simulink model "Linear_model_Kalman_Bucy"  (R2025b)
settings: Solver=VariableStepAuto  StartTime=0.0  StopTime=10.0  RelTol=1e-3
values from neighbouring files (symbols this model uses):
  A1 = [0, 1; 0, 0]    [ABCDmatrixes_for_linear.m]    (also in drone_model_parameters.mat = [0  1; 0  0]; kalman_observer_linear_Q9_RUN_THIS.m)
  A2 = [0, 0, 1, 0; 0, 0, 0, 1; 0, g, 0, 0; 0, 0, 0, 0]    [ABCDmatrixes_for_linear.m]    (also in drone_model_parameters.mat = [0 0 0 0 0 0 9.81 0 1 0 0 0 ... (16 elements, 4x4)]; kalman_observer_linear_Q9_RUN_THIS.m)
  A3 = [0, 0, 1, 0; 0, 0, 0, 1; 0, -g, 0, 0; 0, 0, 0, 0]    [ABCDmatrixes_for_linear.m]    (also in drone_model_parameters.mat = [0 0 0 0 0 0 -9.81 0 1 0 0 0 ... (16 elements, 4x4)]; kalman_observer_linear_Q9_RUN_THIS.m)
  A4 = [0, 1; 0, 0]    [ABCDmatrixes_for_linear.m]    (also in drone_model_parameters.mat = [0  1; 0  0]; kalman_observer_linear_Q9_RUN_THIS.m)
  B1 = [0; 1/m]    [ABCDmatrixes_for_linear.m]    (also in drone_model_parameters.mat = [0 15.873015873]; kalman_observer_linear_Q9_RUN_THIS.m)
  B2 = [0; 0; 0; 1/J11]    [ABCDmatrixes_for_linear.m]    (also in drone_model_parameters.mat = [0 0 0 17156.7786432]; kalman_observer_linear_Q9_RUN_THIS.m)
  B3 = [0; 0; 0; 1/J22]    [ABCDmatrixes_for_linear.m]    (also in drone_model_parameters.mat = [0 0 0 13948.7522841]; kalman_observer_linear_Q9_RUN_THIS.m)
  B4 = [0; 1/J33]    [ABCDmatrixes_for_linear.m]    (also in drone_model_parameters.mat = [0 33333.3333333]; kalman_observer_linear_Q9_RUN_THIS.m)
  C1 = eye(2)    [ABCDmatrixes_for_linear.m]    (also in drone_model_parameters.mat = [1  0; 0  1]; kalman_observer_linear_Q9_RUN_THIS.m)
  C2 = eye(4)    [ABCDmatrixes_for_linear.m]    (also in drone_model_parameters.mat = [1 0 0 0 0 1 0 0 0 0 1 0 ... (16 elements, 4x4)]; kalman_observer_linear_Q9_RUN_THIS.m)
  C3 = eye(4)    [ABCDmatrixes_for_linear.m]    (also in drone_model_parameters.mat = [1 0 0 0 0 1 0 0 0 0 1 0 ... (16 elements, 4x4)]; kalman_observer_linear_Q9_RUN_THIS.m)
  C4 = eye(2)    [ABCDmatrixes_for_linear.m]    (also in drone_model_parameters.mat = [1  0; 0  1]; kalman_observer_linear_Q9_RUN_THIS.m)
  K1 = [0.567 0.2646]    [drone_model_parameters.mat]    (also in kalman_observer_linear_Q9_RUN_THIS.m = place(A1, B1, poles1); lqr_servo_controller.m = K1_lqr(1:2))
  K2 = [0.00422225922936 0.00948429792 0.00292221406239 0.001282292]    [drone_model_parameters.mat]    (also in kalman_observer_linear_Q9_RUN_THIS.m = place(A2, B2, poles2); lqr_servo_controller.m = K2_lqr(1:4))
  K3 = [-0.00519332234862 0.01166555952 -0.00359428419083 0.001577202]    [drone_model_parameters.mat]    (also in kalman_observer_linear_Q9_RUN_THIS.m = place(A3, B3, poles3); lqr_servo_controller.m = K3_lqr(1:4))
  K4 = [0.00015 0.000135]    [drone_model_parameters.mat]    (also in kalman_observer_linear_Q9_RUN_THIS.m = place(A4, B4, poles4); lqr_servo_controller.m = K4_lqr(1:2))
  ki1 = 0.567    [drone_model_parameters.mat]    (also in kalman_observer_linear_Q9_RUN_THIS.m = prefilter(A1, B1, C1(1,:), K1); lqr_servo_controller.m = -K1_lqr(3))
  ki2 = 0.00422225922936    [drone_model_parameters.mat]    (also in kalman_observer_linear_Q9_RUN_THIS.m = prefilter(A2, B2, C2(1,:), K2); lqr_servo_controller.m = -K2_lqr(5))
  ki3 = -0.00519332234862    [drone_model_parameters.mat]    (also in kalman_observer_linear_Q9_RUN_THIS.m = prefilter(A3, B3, C3(1,:), K3); lqr_servo_controller.m = -K3_lqr(5))
  ki4 = 0.00015    [drone_model_parameters.mat]    (also in kalman_observer_linear_Q9_RUN_THIS.m = prefilter(A4, B4, C4(1,:), K4); lqr_servo_controller.m = -K4_lqr(3))
  L1 = [7.45658027326  0.497973338958; 0.0505189943149  7.39637645576]    [drone_model_parameters.mat]
  L2 = [1.45150777342 2.3802958397e-05 0.00454213306172 -1.52026813527e-09 0.0292749657214 29.2123228098 7.26957664981 0.00232988214846 0.87651500602 1.14062573329 10.208521833 2.76371424964e-05 ... (16 elements, 4x4)]    [drone_model_parameters.mat]
  L3 = [1.11002532922 -8.8269645689e-06 0.00273068540644 1.79452583191e-09 -0.0248011961907 27.5933010049 -7.19451191698 0.00571707644971 0.901052348557 -0.844925554559 10.0312929821 -6.86940481085e-05 ... (16 elements, 4x4)]    [drone_model_parameters.mat]
  L4 = [1.61563059299  0.880343962343; 0.000162624550244  11.8866600113]    [drone_model_parameters.mat]
  noise_P_lat = [0.009 0.003 0.002 1e-05]    [drone_model_parameters.mat]    (also in kalman_observer_linear_Q9_RUN_THIS.m = [var_P_r2,  var_P_th1, var_P_v2,  var_P_om1] * Ts)
  noise_P_lon = [0.009 0.002 0.002 1e-05]    [drone_model_parameters.mat]    (also in kalman_observer_linear_Q9_RUN_THIS.m = [var_P_r1,  var_P_th2, var_P_v1,  var_P_om2] * Ts)
  noise_P_vert = [0.001 0.0001]    [drone_model_parameters.mat]    (also in kalman_observer_linear_Q9_RUN_THIS.m = [var_P_r3,  var_P_v3]  * Ts)
  noise_P_yaw = [0.001 1e-05]    [drone_model_parameters.mat]    (also in kalman_observer_linear_Q9_RUN_THIS.m = [var_P_th3, var_P_om3] * Ts)
  phi_ref = 1    [drone_model_parameters.mat]    (also in kalman_observer_linear_Q9_RUN_THIS.m)
  Ts = 0.01    [drone_model_parameters.mat]    (also in kalman_observer_linear_Q9_RUN_THIS.m)
  x0_1 = [0 0]    [drone_model_parameters.mat]    (also in kalman_observer_linear_Q9_RUN_THIS.m = [0; 0])
  x0_2 = [0 0 0 0]    [drone_model_parameters.mat]    (also in kalman_observer_linear_Q9_RUN_THIS.m = [0; 0; 0; 0])
  x0_3 = [0 0 0 0]    [drone_model_parameters.mat]    (also in kalman_observer_linear_Q9_RUN_THIS.m = [0; 0; 0; 0])
  x0_4 = [0 0]    [drone_model_parameters.mat]    (also in kalman_observer_linear_Q9_RUN_THIS.m = [0; 0])
  x0_obs1 = [0 0]    [drone_model_parameters.mat]    (also in kalman_observer_linear_Q9_RUN_THIS.m = [0; 0])
  x0_obs2 = [0 0 0 0]    [drone_model_parameters.mat]    (also in kalman_observer_linear_Q9_RUN_THIS.m = [0; 0; 0; 0])
  x0_obs3 = [0 0 0 0]    [drone_model_parameters.mat]    (also in kalman_observer_linear_Q9_RUN_THIS.m = [0; 0; 0; 0])
  x0_obs4 = [0 0]    [drone_model_parameters.mat]    (also in kalman_observer_linear_Q9_RUN_THIS.m = [0; 0])
  x_ref = 4    [drone_model_parameters.mat]    (also in kalman_observer_linear_Q9_RUN_THIS.m)
  y_ref = 4    [drone_model_parameters.mat]    (also in kalman_observer_linear_Q9_RUN_THIS.m)
  z_ref = 4    [drone_model_parameters.mat]    (also in kalman_observer_linear_Q9_RUN_THIS.m)
libraries: simulink x8
settings Model: Creator=joaom  LastModifiedBy=pepev
settings DataIOCC: SaveFormat=Array

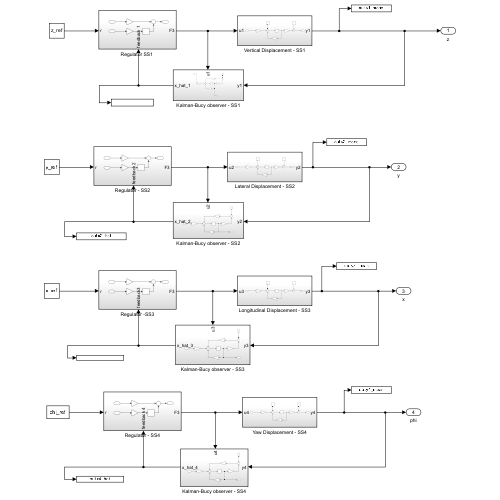
[thumbnail: Simulink's stored preview of the top-level diagram]
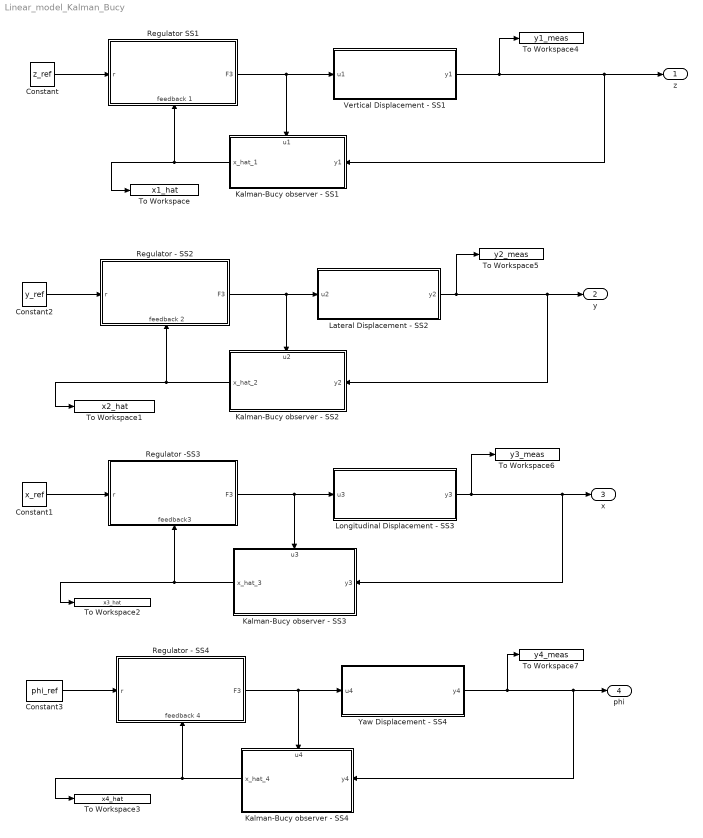
== system Linear_model_Kalman_Bucy ==
  Constant : Constant  Value=z_ref
  Constant1 : Constant  Value=x_ref
  Constant2 : Constant  Value=y_ref
  Constant3 : Constant  Value=phi_ref
  Kalman-Bucy observer - SS1 : Subsystem
      settings: PortSchema="{\"entries\":[{\"content\":{\"sides\":[{\"content\":{\"connectorIds\":[\"Out1\"]},\"type\":\"ConnectorPlacement.EquallySpacedRectSide\",\"uuid\":\"3a34d9e3-ef6b-4e0e-ad1c-a8e9abb9cb50\"},{\"content\":{\"connectorIds\":[\"In2\"],\"side\":\"RIGHT\"},\"type\":\"ConnectorPlacement.EquallySpacedRectSide\",\"uuid\":\"1b685036-9c62-4d8c-a792-6e44f47fda20\"},{\"content\":{\"connectorIds\":[\"In1\"],\"side\":\"TOP\"},\"type\":\"ConnectorPlacement.EquallySpacedRectSide\",\"uuid\":\"5c00f917-5739-44a5-95b0-e7bd6f61a97f\"}]},\"type\":\"ConnectorPlacement.EquallySpacedConnector\",\"uuid\":\"e365f2b2-c96f-4048-9751-de98e4d7538e\"}],\"packageUris\":[\"http://schema.mathworks.com/mf0/Connector/R2020b\"],\"version\":\"1.0\"}"
  Kalman-Bucy observer - SS2 : Subsystem
      settings: PortSchema="{\"entries\":[{\"content\":{\"sides\":[{\"content\":{\"connectorIds\":[\"Out1\"]},\"type\":\"ConnectorPlacement.EquallySpacedRectSide\",\"uuid\":\"3a34d9e3-ef6b-4e0e-ad1c-a8e9abb9cb50\"},{\"content\":{\"connectorIds\":[\"In2\"],\"side\":\"RIGHT\"},\"type\":\"ConnectorPlacement.EquallySpacedRectSide\",\"uuid\":\"1b685036-9c62-4d8c-a792-6e44f47fda20\"},{\"content\":{\"connectorIds\":[\"In1\"],\"side\":\"TOP\"},\"type\":\"ConnectorPlacement.EquallySpacedRectSide\",\"uuid\":\"5c00f917-5739-44a5-95b0-e7bd6f61a97f\"}]},\"type\":\"ConnectorPlacement.EquallySpacedConnector\",\"uuid\":\"e365f2b2-c96f-4048-9751-de98e4d7538e\"}],\"packageUris\":[\"http://schema.mathworks.com/mf0/Connector/R2020b\"],\"version\":\"1.0\"}"
  Kalman-Bucy observer - SS3 : Subsystem
      settings: PortSchema="{\"entries\":[{\"content\":{\"sides\":[{\"content\":{\"connectorIds\":[\"Out1\"]},\"type\":\"ConnectorPlacement.EquallySpacedRectSide\",\"uuid\":\"3a34d9e3-ef6b-4e0e-ad1c-a8e9abb9cb50\"},{\"content\":{\"connectorIds\":[\"In2\"],\"side\":\"RIGHT\"},\"type\":\"ConnectorPlacement.EquallySpacedRectSide\",\"uuid\":\"1b685036-9c62-4d8c-a792-6e44f47fda20\"},{\"content\":{\"connectorIds\":[\"In1\"],\"side\":\"TOP\"},\"type\":\"ConnectorPlacement.EquallySpacedRectSide\",\"uuid\":\"5c00f917-5739-44a5-95b0-e7bd6f61a97f\"}]},\"type\":\"ConnectorPlacement.EquallySpacedConnector\",\"uuid\":\"e365f2b2-c96f-4048-9751-de98e4d7538e\"}],\"packageUris\":[\"http://schema.mathworks.com/mf0/Connector/R2020b\"],\"version\":\"1.0\"}"
  Kalman-Bucy observer - SS4 : Subsystem
      settings: PortSchema="{\"entries\":[{\"content\":{\"sides\":[{\"content\":{\"connectorIds\":[\"Out1\"]},\"type\":\"ConnectorPlacement.EquallySpacedRectSide\",\"uuid\":\"3a34d9e3-ef6b-4e0e-ad1c-a8e9abb9cb50\"},{\"content\":{\"connectorIds\":[\"In2\"],\"side\":\"RIGHT\"},\"type\":\"ConnectorPlacement.EquallySpacedRectSide\",\"uuid\":\"1b685036-9c62-4d8c-a792-6e44f47fda20\"},{\"content\":{\"connectorIds\":[\"In1\"],\"side\":\"TOP\"},\"type\":\"ConnectorPlacement.EquallySpacedRectSide\",\"uuid\":\"5c00f917-5739-44a5-95b0-e7bd6f61a97f\"}]},\"type\":\"ConnectorPlacement.EquallySpacedConnector\",\"uuid\":\"e365f2b2-c96f-4048-9751-de98e4d7538e\"}],\"packageUris\":[\"http://schema.mathworks.com/mf0/Connector/R2020b\"],\"version\":\"1.0\"}"
  Lateral Displacement - SS2 : Subsystem
  Longitudinal Displacement - SS3 : Subsystem
  Regulator - SS2 : Subsystem
      settings: PortSchema="{\"entries\":[{\"content\":{\"sides\":[{\"content\":{\"connectorIds\":[\"In1\"]},\"type\":\"ConnectorPlacement.EquallySpacedRectSide\",\"uuid\":\"b3654a7f-5063-48c0-9b36-91e0db63b0ba\"},{\"content\":{\"connectorIds\":[\"Out1\"],\"side\":\"RIGHT\"},\"type\":\"ConnectorPlacement.EquallySpacedRectSide\",\"uuid\":\"218488d6-68f2-41aa-8299-f3fb09ba40d8\"},{\"content\":{\"side\":\"TOP\"},\"type\":\"ConnectorPlacement.EquallySpacedRectSide\",\"uuid\":\"ffca8f5f-99ce-4cfe-b848-505d5918397a\"},{\"content\":{\"connectorIds\":[\"In2\"],\"side\":\"BOTTOM\"},\"type\":\"ConnectorPlacement.EquallySpacedRectSide\",\"uuid\":\"0ee1b0b7-fa1d-4d2f-b721-1db90edeb8b7\"}]},\"type\":\"ConnectorPlacement.EquallySpacedConnector\",\"uuid\":\"97e1b17e-acc2-4e54-bcf8-8316abbe6834\"}],\"packageUris\":[\"http://schema.mathworks.com/mf0/Connector/R2020b\"],\"version\":\"1.0\"}"
  Regulator - SS4 : Subsystem
      settings: PortSchema="{\"entries\":[{\"content\":{\"sides\":[{\"content\":{\"connectorIds\":[\"In1\"]},\"type\":\"ConnectorPlacement.EquallySpacedRectSide\",\"uuid\":\"b3654a7f-5063-48c0-9b36-91e0db63b0ba\"},{\"content\":{\"connectorIds\":[\"Out1\"],\"side\":\"RIGHT\"},\"type\":\"ConnectorPlacement.EquallySpacedRectSide\",\"uuid\":\"218488d6-68f2-41aa-8299-f3fb09ba40d8\"},{\"content\":{\"side\":\"TOP\"},\"type\":\"ConnectorPlacement.EquallySpacedRectSide\",\"uuid\":\"ffca8f5f-99ce-4cfe-b848-505d5918397a\"},{\"content\":{\"connectorIds\":[\"In2\"],\"side\":\"BOTTOM\"},\"type\":\"ConnectorPlacement.EquallySpacedRectSide\",\"uuid\":\"0ee1b0b7-fa1d-4d2f-b721-1db90edeb8b7\"}]},\"type\":\"ConnectorPlacement.EquallySpacedConnector\",\"uuid\":\"97e1b17e-acc2-4e54-bcf8-8316abbe6834\"}],\"packageUris\":[\"http://schema.mathworks.com/mf0/Connector/R2020b\"],\"version\":\"1.0\"}"
  Regulator -SS3 : Subsystem
      settings: PortSchema="{\"entries\":[{\"content\":{\"sides\":[{\"content\":{\"connectorIds\":[\"In1\"]},\"type\":\"ConnectorPlacement.EquallySpacedRectSide\",\"uuid\":\"b3654a7f-5063-48c0-9b36-91e0db63b0ba\"},{\"content\":{\"connectorIds\":[\"Out1\"],\"side\":\"RIGHT\"},\"type\":\"ConnectorPlacement.EquallySpacedRectSide\",\"uuid\":\"218488d6-68f2-41aa-8299-f3fb09ba40d8\"},{\"content\":{\"side\":\"TOP\"},\"type\":\"ConnectorPlacement.EquallySpacedRectSide\",\"uuid\":\"ffca8f5f-99ce-4cfe-b848-505d5918397a\"},{\"content\":{\"connectorIds\":[\"In2\"],\"side\":\"BOTTOM\"},\"type\":\"ConnectorPlacement.EquallySpacedRectSide\",\"uuid\":\"0ee1b0b7-fa1d-4d2f-b721-1db90edeb8b7\"}]},\"type\":\"ConnectorPlacement.EquallySpacedConnector\",\"uuid\":\"97e1b17e-acc2-4e54-bcf8-8316abbe6834\"}],\"packageUris\":[\"http://schema.mathworks.com/mf0/Connector/R2020b\"],\"version\":\"1.0\"}"
  "Regulator SS1 " : Subsystem
      settings: PortSchema="{\"entries\":[{\"content\":{\"sides\":[{\"content\":{\"connectorIds\":[\"In1\"]},\"type\":\"ConnectorPlacement.EquallySpacedRectSide\",\"uuid\":\"b3654a7f-5063-48c0-9b36-91e0db63b0ba\"},{\"content\":{\"connectorIds\":[\"Out1\"],\"side\":\"RIGHT\"},\"type\":\"ConnectorPlacement.EquallySpacedRectSide\",\"uuid\":\"218488d6-68f2-41aa-8299-f3fb09ba40d8\"},{\"content\":{\"side\":\"TOP\"},\"type\":\"ConnectorPlacement.EquallySpacedRectSide\",\"uuid\":\"ffca8f5f-99ce-4cfe-b848-505d5918397a\"},{\"content\":{\"connectorIds\":[\"In2\"],\"side\":\"BOTTOM\"},\"type\":\"ConnectorPlacement.EquallySpacedRectSide\",\"uuid\":\"0ee1b0b7-fa1d-4d2f-b721-1db90edeb8b7\"}]},\"type\":\"ConnectorPlacement.EquallySpacedConnector\",\"uuid\":\"97e1b17e-acc2-4e54-bcf8-8316abbe6834\"}],\"packageUris\":[\"http://schema.mathworks.com/mf0/Connector/R2020b\"],\"version\":\"1.0\"}"
  To Workspace : ToWorkspace  VariableName=x1_hat  SampleTime=-1
  To Workspace1 : ToWorkspace  VariableName=x2_hat  SampleTime=-1
  To Workspace2 : ToWorkspace  VariableName=x3_hat  SampleTime=-1
  To Workspace3 : ToWorkspace  VariableName=x4_hat  SampleTime=-1
  To Workspace4 : ToWorkspace  VariableName=y1_meas  SampleTime=-1
  To Workspace5 : ToWorkspace  VariableName=y2_meas  SampleTime=-1
  To Workspace6 : ToWorkspace  VariableName=y3_meas  SampleTime=-1
  To Workspace7 : ToWorkspace  VariableName=y4_meas  SampleTime=-1
  Vertical Displacement - SS1 : Subsystem
  Yaw Displacement - SS4 : Subsystem
  z : Outport
  y : Outport  Port=2
  x : Outport  Port=3
  phi : Outport  Port=4
  wires:
  Constant/1 -> "Regulator SS1 "/1(r)
  "Regulator SS1 "/1(F3) -> Kalman-Bucy observer - SS1/1(u1), Vertical Displacement - SS1/1(u1)
  Constant2/1 -> Regulator - SS2/1(r)
  Regulator - SS2/1(F3) -> Kalman-Bucy observer - SS2/1(u2), Lateral Displacement - SS2/1(u2)
  Constant1/1 -> Regulator -SS3/1(r)
  Regulator -SS3/1(F3) -> Longitudinal Displacement - SS3/1(u3), Kalman-Bucy observer - SS3/1(u3)
  Yaw Displacement - SS4/1(y4) -> To Workspace7/1, Kalman-Bucy observer - SS4/2(y4), phi/1
  Constant3/1 -> Regulator - SS4/1(r)
  Regulator - SS4/1(F3) -> Kalman-Bucy observer - SS4/1(u4), Yaw Displacement - SS4/1(u4)
  Kalman-Bucy observer - SS1/1(x_hat_1) -> To Workspace/1, "Regulator SS1 "/2(feedback 1)
  Kalman-Bucy observer - SS3/1(x_hat_3) -> To Workspace2/1, Regulator -SS3/2(feedback3)
  Kalman-Bucy observer - SS4/1(x_hat_4) -> To Workspace3/1, Regulator - SS4/2(feedback 4)
  Kalman-Bucy observer - SS2/1(x_hat_2) -> Regulator - SS2/2(feedback 2), To Workspace1/1
  Vertical Displacement - SS1/1(y1) -> Kalman-Bucy observer - SS1/2(y1), z/1, To Workspace4/1
  Lateral Displacement - SS2/1(y2) -> To Workspace5/1, Kalman-Bucy observer - SS2/2(y2), y/1
  Longitudinal Displacement - SS3/1(y3) -> To Workspace6/1, Kalman-Bucy observer - SS3/2(y3), x/1

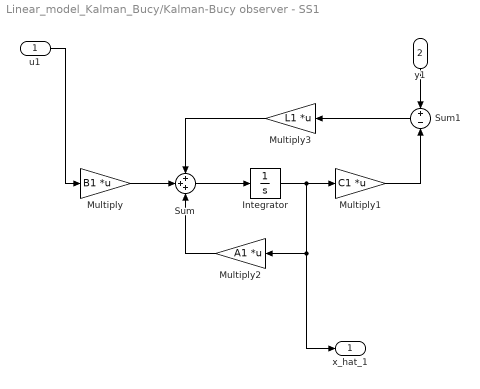
== system Linear_model_Kalman_Bucy/Kalman-Bucy observer - SS1 ==
  u1 : Inport
  y1 : Inport  Port=2
  Integrator : Integrator  InitialCondition=x0_obs1
  Multiply : Gain  Gain=B1  Multiplication=Matrix(K*u)
  Multiply1 : Gain  Gain=C1  Multiplication=Matrix(K*u)
  Multiply2 : Gain  Gain=A1  Multiplication=Matrix(K*u)
  Multiply3 : Gain  Gain=L1  Multiplication=Matrix(K*u)
  Sum : Sum  Inputs=+++
  Sum1 : Sum  Inputs=+|-
  x_hat_1 : Outport
  wires:
  Multiply2/1 -> Sum/3
  Sum/1 -> Integrator/1
  Integrator/1 -> x_hat_1/1, Multiply2/1, Multiply1/1
  u1/1 -> Multiply/1
  Multiply3/1 -> Sum/1
  Multiply/1 -> Sum/2
  Multiply1/1 -> Sum1/2
  y1/1 -> Sum1/1
  Sum1/1 -> Multiply3/1

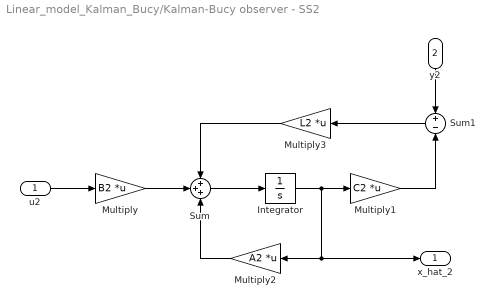
== system Linear_model_Kalman_Bucy/Kalman-Bucy observer - SS2 ==
  u2 : Inport
  y2 : Inport  Port=2
  Integrator : Integrator  InitialCondition=x0_obs2
  Multiply : Gain  Gain=B2  Multiplication=Matrix(K*u)
  Multiply1 : Gain  Gain=C2  Multiplication=Matrix(K*u)
  Multiply2 : Gain  Gain=A2  Multiplication=Matrix(K*u)
  Multiply3 : Gain  Gain=L2  Multiplication=Matrix(K*u)
  Sum : Sum  Inputs=+++
  Sum1 : Sum  Inputs=+|-
  x_hat_2 : Outport
  wires:
  Multiply2/1 -> Sum/3
  Sum/1 -> Integrator/1
  Integrator/1 -> x_hat_2/1, Multiply2/1, Multiply1/1
  u2/1 -> Multiply/1
  Multiply3/1 -> Sum/1
  Multiply/1 -> Sum/2
  Multiply1/1 -> Sum1/2
  y2/1 -> Sum1/1
  Sum1/1 -> Multiply3/1

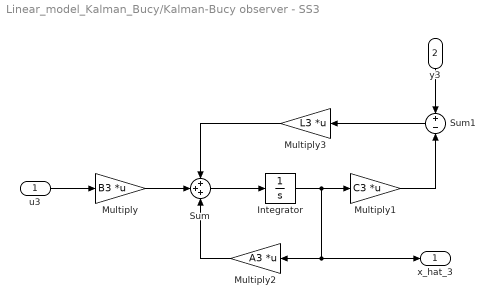
== system Linear_model_Kalman_Bucy/Kalman-Bucy observer - SS3 ==
  u3 : Inport
  y3 : Inport  Port=2
  Integrator : Integrator  InitialCondition=x0_obs3
  Multiply : Gain  Gain=B3  Multiplication=Matrix(K*u)
  Multiply1 : Gain  Gain=C3  Multiplication=Matrix(K*u)
  Multiply2 : Gain  Gain=A3  Multiplication=Matrix(K*u)
  Multiply3 : Gain  Gain=L3  Multiplication=Matrix(K*u)
  Sum : Sum  Inputs=+++
  Sum1 : Sum  Inputs=+|-
  x_hat_3 : Outport
  wires:
  Multiply2/1 -> Sum/3
  Sum/1 -> Integrator/1
  Integrator/1 -> x_hat_3/1, Multiply2/1, Multiply1/1
  u3/1 -> Multiply/1
  Multiply3/1 -> Sum/1
  Multiply/1 -> Sum/2
  Multiply1/1 -> Sum1/2
  y3/1 -> Sum1/1
  Sum1/1 -> Multiply3/1

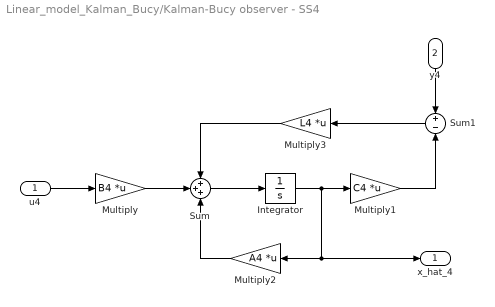
== system Linear_model_Kalman_Bucy/Kalman-Bucy observer - SS4 ==
  u4 : Inport
  y4 : Inport  Port=2
  Integrator : Integrator  InitialCondition=x0_obs4
  Multiply : Gain  Gain=B4  Multiplication=Matrix(K*u)
  Multiply1 : Gain  Gain=C4  Multiplication=Matrix(K*u)
  Multiply2 : Gain  Gain=A4  Multiplication=Matrix(K*u)
  Multiply3 : Gain  Gain=L4  Multiplication=Matrix(K*u)
  Sum : Sum  Inputs=+++
  Sum1 : Sum  Inputs=+|-
  x_hat_4 : Outport
  wires:
  Multiply2/1 -> Sum/3
  Sum/1 -> Integrator/1
  Integrator/1 -> x_hat_4/1, Multiply2/1, Multiply1/1
  u4/1 -> Multiply/1
  Multiply3/1 -> Sum/1
  Multiply/1 -> Sum/2
  Multiply1/1 -> Sum1/2
  y4/1 -> Sum1/1
  Sum1/1 -> Multiply3/1

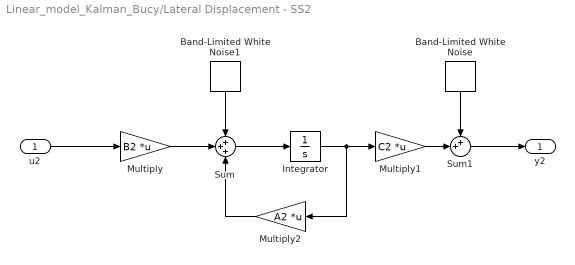
== system Linear_model_Kalman_Bucy/Lateral Displacement - SS2 ==
  u2 : Inport
  Band-Limited White Noise : simulink/Sources/Band-Limited White Noise  Cov=noise_M_lat  Ts=0.01  seed=[50 51 52 53]
  Band-Limited White Noise1 : simulink/Sources/Band-Limited White Noise  Cov=[noise_P_lat]  Ts=0.01  seed=[46 47 48 49]
  Integrator : Integrator  InitialCondition=x0_2
  Multiply : Gain  Gain=B2  Multiplication=Matrix(K*u)
  Multiply1 : Gain  Gain=C2  Multiplication=Matrix(K*u)
  Multiply2 : Gain  Gain=A2  Multiplication=Matrix(K*u)
  Sum : Sum  Inputs=+++
  Sum1 : Sum  Inputs=++|
  y2 : Outport
  wires:
  u2/1 -> Multiply/1
  Multiply/1 -> Sum/2
  Sum/1 -> Integrator/1
  Integrator/1 -> Multiply2/1, Multiply1/1
  Multiply1/1 -> Sum1/2
  Sum1/1 -> y2/1
  Multiply2/1 -> Sum/3
  Band-Limited White Noise/1 -> Sum1/1
  Band-Limited White Noise1/1 -> Sum/1

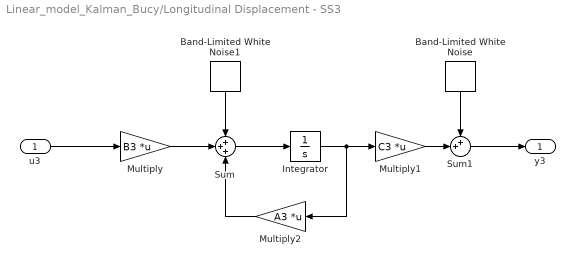
== system Linear_model_Kalman_Bucy/Longitudinal Displacement - SS3 ==
  u3 : Inport
  Band-Limited White Noise : simulink/Sources/Band-Limited White Noise  Cov=noise_M_lon  Ts=0.01  seed=[58 59 60 61]
  Band-Limited White Noise1 : simulink/Sources/Band-Limited White Noise  Cov=[noise_P_lon]  Ts=0.01  seed=[54 55 56 57]
  Integrator : Integrator  InitialCondition=x0_3
  Multiply : Gain  Gain=B3  Multiplication=Matrix(K*u)
  Multiply1 : Gain  Gain=C3  Multiplication=Matrix(K*u)
  Multiply2 : Gain  Gain=A3  Multiplication=Matrix(K*u)
  Sum : Sum  Inputs=+++
  Sum1 : Sum  Inputs=++|
  y3 : Outport
  wires:
  u3/1 -> Multiply/1
  Multiply/1 -> Sum/2
  Sum/1 -> Integrator/1
  Integrator/1 -> Multiply2/1, Multiply1/1
  Multiply1/1 -> Sum1/2
  Sum1/1 -> y3/1
  Multiply2/1 -> Sum/3
  Band-Limited White Noise/1 -> Sum1/1
  Band-Limited White Noise1/1 -> Sum/1

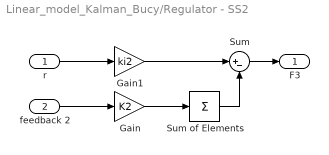
== system Linear_model_Kalman_Bucy/Regulator - SS2 ==
  r : Inport
  feedback 2 : Inport  Port=2
  Gain : Gain  Gain=K2
  Gain1 : Gain  Gain=ki2
  Sum : Sum  Inputs=|+-
  Sum of Elements : Sum  Inputs=+
  F3 : Outport
  wires:
  r/1 -> Gain1/1
  Gain1/1 -> Sum/1
  Sum/1 -> F3/1
  feedback 2/1 -> Gain/1
  Gain/1 -> Sum of Elements/1
  Sum of Elements/1 -> Sum/2

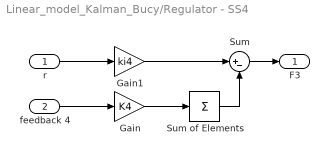
== system Linear_model_Kalman_Bucy/Regulator - SS4 ==
  r : Inport
  feedback 4 : Inport  Port=2
  Gain : Gain  Gain=K4
  Gain1 : Gain  Gain=ki4
  Sum : Sum  Inputs=|+-
  Sum of Elements : Sum  Inputs=+
  F3 : Outport
  wires:
  r/1 -> Gain1/1
  Gain1/1 -> Sum/1
  Sum/1 -> F3/1
  feedback 4/1 -> Gain/1
  Gain/1 -> Sum of Elements/1
  Sum of Elements/1 -> Sum/2

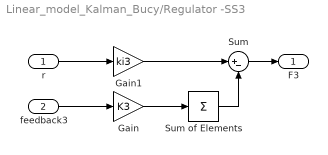
== system Linear_model_Kalman_Bucy/Regulator -SS3 ==
  r : Inport
  feedback3 : Inport  Port=2
  Gain : Gain  Gain=K3
  Gain1 : Gain  Gain=ki3
  Sum : Sum  Inputs=|+-
  Sum of Elements : Sum  Inputs=+
  F3 : Outport
  wires:
  r/1 -> Gain1/1
  Gain1/1 -> Sum/1
  Sum/1 -> F3/1
  feedback3/1 -> Gain/1
  Gain/1 -> Sum of Elements/1
  Sum of Elements/1 -> Sum/2

== system Linear_model_Kalman_Bucy/Regulator SS1  ==
  r : Inport
  feedback 1 : Inport  Port=2
  Gain : Gain  Gain=K1
  Gain1 : Gain  Gain=ki1
  Sum : Sum  Inputs=|+-
  Sum of Elements : Sum  Inputs=+
  F3 : Outport
  wires:
  r/1 -> Gain1/1
  Gain1/1 -> Sum/1
  Sum/1 -> F3/1
  feedback 1/1 -> Gain/1
  Gain/1 -> Sum of Elements/1
  Sum of Elements/1 -> Sum/2

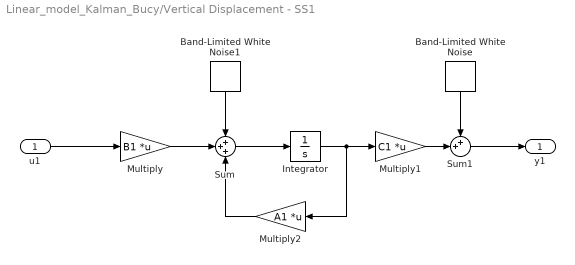
== system Linear_model_Kalman_Bucy/Vertical Displacement - SS1 ==
  u1 : Inport
  Band-Limited White Noise : simulink/Sources/Band-Limited White Noise  Cov=noise_M_vert  Ts=0.01  seed=[44 45]
  Band-Limited White Noise1 : simulink/Sources/Band-Limited White Noise  Cov=[noise_P_vert]  Ts=Ts  seed=[42 43]
  Integrator : Integrator  InitialCondition=x0_1
  Multiply : Gain  Gain=B1  Multiplication=Matrix(K*u)
  Multiply1 : Gain  Gain=C1  Multiplication=Matrix(K*u)
  Multiply2 : Gain  Gain=A1  Multiplication=Matrix(K*u)
  Sum : Sum  Inputs=+++
  Sum1 : Sum  Inputs=++|
  y1 : Outport
  wires:
  u1/1 -> Multiply/1
  Multiply/1 -> Sum/2
  Sum/1 -> Integrator/1
  Integrator/1 -> Multiply2/1, Multiply1/1
  Multiply1/1 -> Sum1/2
  Sum1/1 -> y1/1
  Multiply2/1 -> Sum/3
  Band-Limited White Noise/1 -> Sum1/1
  Band-Limited White Noise1/1 -> Sum/1

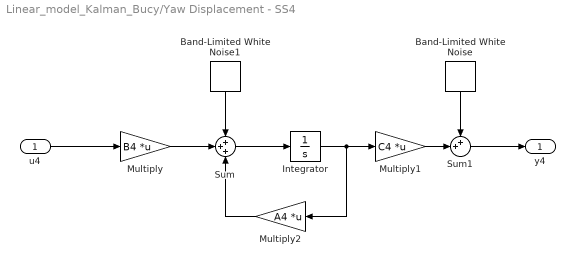
== system Linear_model_Kalman_Bucy/Yaw Displacement - SS4 ==
  u4 : Inport
  Band-Limited White Noise : simulink/Sources/Band-Limited White Noise  Cov=noise_M_yaw  Ts=0.01  seed=[64 65]
  Band-Limited White Noise1 : simulink/Sources/Band-Limited White Noise  Cov=[noise_P_yaw]  Ts=0.01  seed=[62 63]
  Integrator : Integrator  InitialCondition=x0_4
  Multiply : Gain  Gain=B4  Multiplication=Matrix(K*u)
  Multiply1 : Gain  Gain=C4  Multiplication=Matrix(K*u)
  Multiply2 : Gain  Gain=A4  Multiplication=Matrix(K*u)
  Sum : Sum  Inputs=+++
  Sum1 : Sum  Inputs=++|
  y4 : Outport
  wires:
  u4/1 -> Multiply/1
  Multiply/1 -> Sum/2
  Sum/1 -> Integrator/1
  Integrator/1 -> Multiply2/1, Multiply1/1
  Multiply1/1 -> Sum1/2
  Sum1/1 -> y4/1
  Multiply2/1 -> Sum/3
  Band-Limited White Noise/1 -> Sum1/1
  Band-Limited White Noise1/1 -> Sum/1
